simulink model "Project1_wk2"  (R2023b)
settings: Solver=VariableStepAuto  StartTime=0.0  StopTime=10.0  RelTol=1e-3
values from neighbouring files (symbols this model uses):
  A = A_a(2)    [Project1.m]    (also in Project1_and_graphing.m; Project1_and_graphing_plz_check.m; Project1_week1.m = 4; Project1_week2.m = [0, 100])
  b = b_a(q)    [Project1.m]    (also in Project1_and_graphing.m; Project1_and_graphing_plz_check.m; Project1_week1.m = 1; Project1_week2.m = [10, 0.1])
  freq = freq_a(p)    [Project1.m]    (also in Project1_and_graphing.m; Project1_and_graphing_plz_check.m)
  J = J_a(r)    [Project1.m]    (also in Project1_and_graphing.m; Project1_and_graphing_plz_check.m; Project1_week1.m = 1; Project1_week2.m = [100, 0.01])
  sin_check = sin_check_a(k)    [Project1.m]    (also in Project1_and_graphing.m; Project1_and_graphing_plz_check.m)
undefined symbols (not defined in the file or in its folder): act
settings Model: Creator=kkern  LastModifiedBy=kkern

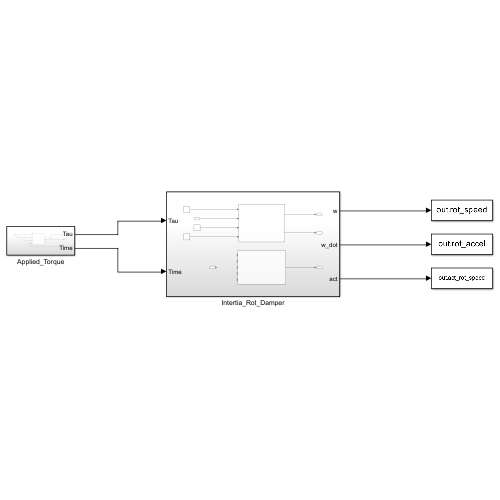
[thumbnail: Simulink's stored preview of the top-level diagram]
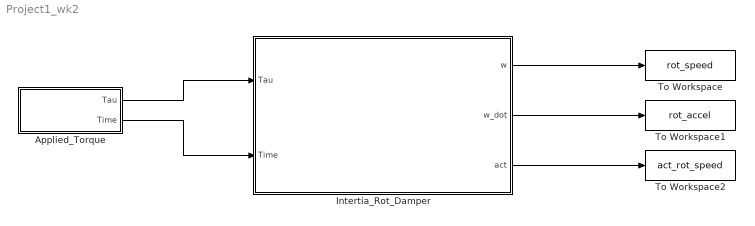
== system Project1_wk2 ==
  Applied_Torque : Subsystem
  Intertia_Rot_Damper : Subsystem
  To Workspace : ToWorkspace  VariableName=rot_speed  SaveFormat=Timeseries  SampleTime=-1
  To Workspace1 : ToWorkspace  VariableName=rot_accel  SaveFormat=Timeseries  SampleTime=-1
  To Workspace2 : ToWorkspace  VariableName=act_rot_speed  SaveFormat=Timeseries  SampleTime=-1
  wires:
  Applied_Torque/1(Tau) -> Intertia_Rot_Damper/1(Tau)
  Applied_Torque/2(Time) -> Intertia_Rot_Damper/2(Time)
  Intertia_Rot_Damper/1(w) -> To Workspace/1
  Intertia_Rot_Damper/2(w_dot) -> To Workspace1/1
  Intertia_Rot_Damper/3(act) -> To Workspace2/1

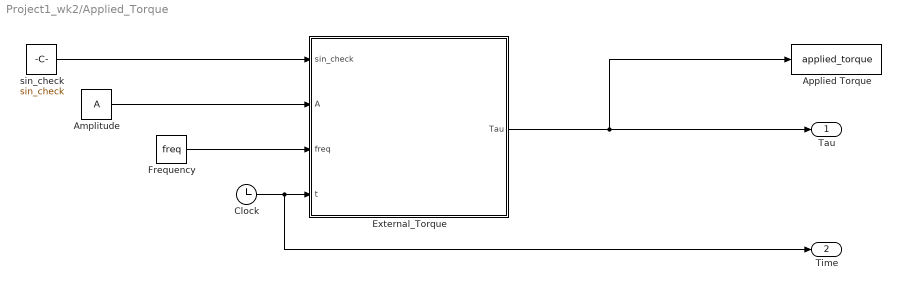
== system Project1_wk2/Applied_Torque ==
  Amplitude : Constant  Value=A
  Applied Torque : ToWorkspace  VariableName=applied_torque  SaveFormat=Timeseries  SampleTime=-1
  Clock : Clock
      settings: Decimation=25
  External_Torque : MATLAB Function  TreatAsAtomicUnit=on
  Frequency : Constant  Value=freq
  sin_check : Constant  Value=sin_check
  Tau : Outport
  Time : Outport  Port=2
  wires:
  Frequency/1 -> External_Torque/3(freq)
  sin_check/1 -> External_Torque/1(sin_check)
  Amplitude/1 -> External_Torque/2(A)
  Clock/1 -> Time/1, External_Torque/4(t)
  External_Torque/1(Tau) -> Tau/1, Applied Torque/1

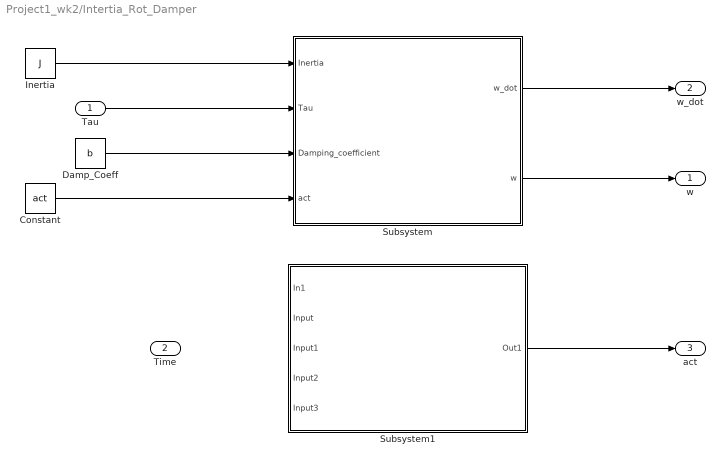
== system Project1_wk2/Intertia_Rot_Damper ==
  Tau : Inport
  Time : Inport  Port=2
  Constant : Constant  Value=act
  Damp_Coeff : Constant  Value=b
  Inertia : Constant  Value=J
  Subsystem : Subsystem
  Subsystem1 : Subsystem
  w : Outport
  w_dot : Outport  Port=2
  act : Outport  Port=3
  wires:
  Subsystem/2(w) -> w/1
  Subsystem/1(w_dot) -> w_dot/1
  Tau/1 -> Subsystem/2(Tau)
  Inertia/1 -> Subsystem/1(Inertia)
  Constant/1 -> Subsystem/4(act)
  Damp_Coeff/1 -> Subsystem/3(Damping_coefficient)
  Subsystem1/1(Out1) -> act/1

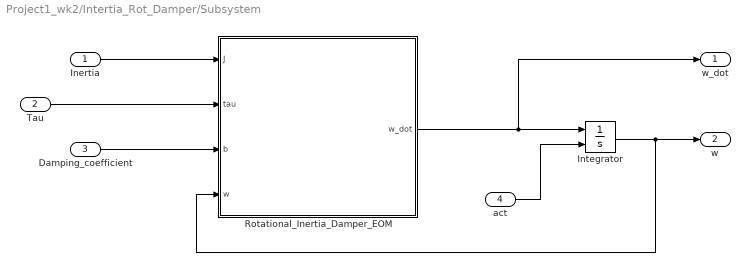
== system Project1_wk2/Intertia_Rot_Damper/Subsystem ==
  Inertia : Inport
  Tau : Inport  Port=2
  Damping_coefficient : Inport  Port=3
  act : Inport  Port=4
  Integrator : Integrator  InitialConditionSource=external
  Rotational_Inertia_Damper_EOM : MATLAB Function  TreatAsAtomicUnit=on
  w_dot : Outport
  w : Outport  Port=2
  wires:
  Integrator/1 -> Rotational_Inertia_Damper_EOM/4(w), w/1
  Inertia/1 -> Rotational_Inertia_Damper_EOM/1(J)
  act/1 -> Integrator/2
  Rotational_Inertia_Damper_EOM/1(w_dot) -> w_dot/1, Integrator/1
  Tau/1 -> Rotational_Inertia_Damper_EOM/2(tau)
  Damping_coefficient/1 -> Rotational_Inertia_Damper_EOM/3(b)

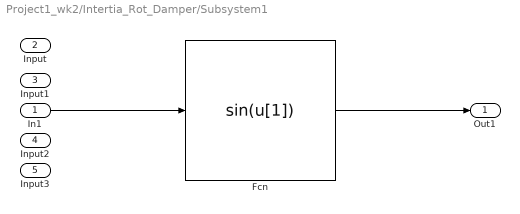
== system Project1_wk2/Intertia_Rot_Damper/Subsystem1 ==
  In1 : Inport
  Input : Inport  Port=2
  Input1 : Inport  Port=3
  Input2 : Inport  Port=4
  Input3 : Inport  Port=5
  Fcn : Fcn
  Out1 : Outport
  wires:
  In1/1 -> Fcn/1
  Fcn/1 -> Out1/1

== matlab function Project1_wk2/Intertia_Rot_Damper/Subsystem/Rotational_Inertia_Damper_EOM ==
  data: J input; tau input; w_dot output; b input; w input
function w_dot = fcn(J, tau, b, w)
% Recall EOM: J*w_dot = tau_applied - tau_damped
tau_damped = b*w;
w_dot = (1/J)*(tau - tau_damped);
end

== matlab function Project1_wk2/Applied_Torque/External_Torque ==
  data: sin_check input; Tau output; A input; freq input; t input
function Tau = fcn(sin_check, A, freq, t)

if (sin_check == 0)
    Tau = A;

else 
    Tau = A*sin(freq*t)
end
